simulink model "opti_debug"  (R2023a)
settings: Solver=FixedStepAuto  StartTime=0.0  StopTime=mdl.rt  RelTol=1e-3
values from neighbouring files (symbols this model uses):
  archived_Eul_XYZ = rst_Eul_XYZ.signals.values    [s4_run.m]    (also in step4_run_v1.m)
  archived_p_raw = rst_p_raw.signals.values    [s4_run.m]    (also in step4_run_v1.m)
  ctr = make_ext_tor_observer(rsim, mdl, ctr)    [s1_setup.m]    (also in setup_controller_with_functions.m = make_controller(); step1_setup.m; step1_setup_v1.m)
  ctr2 = ctr    [s1_setup.m]    (also in step1_setup.m; step1_setup_v1.m)
  lut = gen_lut    [s1_setup.m]    (also in thrust2voltage_lut_20230809.mat = ; thrust2voltage_lut_20230829.mat = )
  mdl = make_model(mdl,rsim)    [s1_setup.m]    (also in setup_controller_with_functions.m = make_model(flight_time); step1_setup.m; step1_setup_v1.m = make_model(flight_time,rsim))
  rbt = make_robot    [s1_setup.m]    (also in setup_controller_with_functions.m = make_robot(); step1_setup.m; step1_setup_v1.m)
  rbt2 = rbt    [s1_setup.m]    (also in step1_setup.m; step1_setup_v1.m)
  rsim = make_robot_simulation()    [setup_controller_with_functions.m]    (also in step1_setup_v1.m = make_simulation(rbt,mdl,rsim))
  sen = make_sensor(mdl,rsim)    [s1_setup.m]
  som = make_somersault(mdl, rsim)    [s1_setup.m]    (also in step1_setup.m)
  Time = logsout.LiveStreamSignals.getElement('voltage').Values.Time    [old_step3_run_controller_v3.m]    (also in post_identify_actuation_response.m = yout(:,1); post_thrust_torque_coefficients.m = yout(:,1))
  traj = make_trajectory(ctr, mdl, rsim)    [s1_setup.m]    (also in step1_setup.m)
undefined symbols (not defined in the file or in its folder): DiscIntNeverNeededParam, Discrete, Standard_Devices, UDP_Protocol
libraries: simulink x27, dspfdesign x12, robotcorelib x7, sldrtlib x7, slrealtimeloglib x1, shared6dof x1, dspsrcs4 x1, uavutilslib x1, ctrlSharedLib x1, dspmathops x1
(part 4 of 4)

== system opti_debug/Signal generater/signal generator1/signal generator 3/get max voltage/SIgnalForRamp_binary ==
  note: Should output 1 or -1,
      | so signal ramps UP to 1
      | or DOWN to 0.
  In1 : Inport
  Add : Sum  Inputs=+-
  Compare To Zero : simulink/Logic and Bit Operations/Compare To Zero  relop=>  OutDataTypeStr=uint8  ZeroCross=off
  Constant : Constant
  Data Type Conversion : DataTypeConversion  OutDataTypeStr=double  SaturateOnIntegerOverflow=off  RndMeth=Floor
  Gain : Gain  Gain=2
  Out1 : Outport
  wires:
  In1/1 -> Compare To Zero/1
  Compare To Zero/1 -> Data Type Conversion/1
  Gain/1 -> Add/1
  Constant/1 -> Add/2
  Add/1 -> Out1/1
  Data Type Conversion/1 -> Gain/1

== system opti_debug/Signal generater/signal generator1/signal generator 3/square root of sine wave/Subsystem1 ==
  cos wave : Inport
  new_amplitude : Inport  Port=2
  Delay : Delay  DelayLength=1  InitialCondition=0
  Delay1 : Delay  InitialCondition=[0,0]
  Delay2 : Delay  DelayLength=1  InitialCondition=0
  MATLAB Function : MATLAB Function  TreatAsAtomicUnit=on  SystemSampleTime=mdl.T_high
  output : Outport
  wires:
  cos wave/1 -> Delay1/1, Delay/1, MATLAB Function/1(u1)
  MATLAB Function/1(output) -> output/1, Delay2/1
  Delay/1 -> MATLAB Function/2(u2)
  Delay2/1 -> MATLAB Function/5(old_amplitude)
  Delay1/1 -> MATLAB Function/3(u3)
  new_amplitude/1 -> MATLAB Function/4(new_amplitude)

== system opti_debug/Signal generater/signal generator1/signal generator 4/get max voltage/SIgnalForRamp_binary ==
  note: Should output 1 or -1,
      | so signal ramps UP to 1
      | or DOWN to 0.
  In1 : Inport
  Add : Sum  Inputs=+-
  Compare To Zero : simulink/Logic and Bit Operations/Compare To Zero  relop=>  OutDataTypeStr=uint8  ZeroCross=off
  Constant : Constant
  Data Type Conversion : DataTypeConversion  OutDataTypeStr=double  SaturateOnIntegerOverflow=off  RndMeth=Floor
  Gain : Gain  Gain=2
  Out1 : Outport
  wires:
  In1/1 -> Compare To Zero/1
  Compare To Zero/1 -> Data Type Conversion/1
  Gain/1 -> Add/1
  Constant/1 -> Add/2
  Add/1 -> Out1/1
  Data Type Conversion/1 -> Gain/1

== system opti_debug/Signal generater/signal generator1/signal generator 4/square root of sine wave/Subsystem1 ==
  cos wave : Inport
  new_amplitude : Inport  Port=2
  Delay : Delay  DelayLength=1  InitialCondition=0
  Delay1 : Delay  InitialCondition=[0,0]
  Delay2 : Delay  DelayLength=1  InitialCondition=0
  MATLAB Function : MATLAB Function  TreatAsAtomicUnit=on  SystemSampleTime=mdl.T_high
  output : Outport
  wires:
  cos wave/1 -> Delay1/1, Delay/1, MATLAB Function/1(u1)
  MATLAB Function/1(output) -> output/1, Delay2/1
  Delay/1 -> MATLAB Function/2(u2)
  Delay2/1 -> MATLAB Function/5(old_amplitude)
  Delay1/1 -> MATLAB Function/3(u3)
  new_amplitude/1 -> MATLAB Function/4(new_amplitude)

== matlab function opti_debug/Motor thrust to voltage mapping/Subsystem/MATLAB Function ==
  data: t input; enable output; mdl parameter
function enable = fcn(t, mdl)

if t > mdl.i_delay && t < (mdl.i_delay + mdl.flight_time)
    enable = 1;
else
    enable = 0;
end

end

== matlab function opti_debug/Archived data for rerun/MATLAB Function1 ==
  data: t input; y output; archived_data_ready parameter
function y = fcn(t,archived_data_ready)

t = floor(t);
y = archived_data_ready(t,1);

end

== matlab function opti_debug/Archived data for rerun/MATLAB Function2 ==
  data: t input; y output; archived_p_raw parameter; archived_Eul_XYZ parameter
function y = fcn(t,archived_p_raw,archived_Eul_XYZ)

y = zeros(6,1);

t = floor(t);
y(1:3,1) = archived_p_raw(t,1:3)';
y(4:6,1) = archived_Eul_XYZ(t,1:3)';

end

== matlab function opti_debug/Control scheme/attitude and thrust controller/Subsystem/MATLAB Function ==
  data: time input; en_int output; ctr parameter; mdl parameter
function en_int = fcn(time, ctr, mdl)

    if ctr.takeoff.en
        wait_time = ctr.takeoff.time;
    else
        wait_time = 0;
    end
    
    if time > (mdl.i_delay + wait_time) && ctr.integral.en
        en_int = 1;
    else 
        en_int = 0;
    end

end

== matlab function opti_debug/Signal generater/signal generator1/signal generator 1/square root of sine wave/Subsystem1/MATLAB Function ==
  data: u1 input; output output; u2 input; u3 input; new_amplitude input; old_amplitude input
function output  = fcn(u1, u2, u3, new_amplitude, old_amplitude)

if u2 < u1 && u2 < u3
    output = new_amplitude;
else
    output = old_amplitude;
end

    
end

== matlab function opti_debug/Signal generater/signal generator1/signal generator 2/square root of sine wave/Subsystem1/MATLAB Function ==
  data: u1 input; output output; u2 input; u3 input; new_amplitude input; old_amplitude input
function output  = fcn(u1, u2, u3, new_amplitude, old_amplitude)

if u2 < u1 && u2 < u3
    output = new_amplitude;
else
    output = old_amplitude;
end

    
end

== matlab function opti_debug/Signal generater/signal generator1/signal generator 3/square root of sine wave/Subsystem1/MATLAB Function ==
  data: u1 input; output output; u2 input; u3 input; new_amplitude input; old_amplitude input
function output  = fcn(u1, u2, u3, new_amplitude, old_amplitude)

if u2 < u1 && u2 < u3
    output = new_amplitude;
else
    output = old_amplitude;
end

    
end

== matlab function opti_debug/Signal generater/signal generator1/signal generator 4/square root of sine wave/Subsystem1/MATLAB Function ==
  data: u1 input; output output; u2 input; u3 input; new_amplitude input; old_amplitude input
function output  = fcn(u1, u2, u3, new_amplitude, old_amplitude)

if u2 < u1 && u2 < u3
    output = new_amplitude;
else
    output = old_amplitude;
end

    
end

== matlab function opti_debug/State filters/IMU orientation/Subsystem2/Rotation Matrix ==
  data: euler_angles input; R output
function R = fcn(euler_angles)
%#codegen

eu_x = euler_angles(1);
eu_y = euler_angles(2);
eu_z = euler_angles(3);

R = [cos(eu_y)*cos(eu_z); -cos(eu_y)*sin(eu_z); sin(eu_y); ...
    cos(eu_x)*sin(eu_z)+sin(eu_x)*sin(eu_y)*cos(eu_z); cos(eu_x)*cos(eu_z)-sin(eu_x)*sin(eu_y)*sin(eu_z); -sin(eu_x)*cos(eu_y); ...
    sin(eu_x)*sin(eu_z)-cos(eu_x)*sin(eu_y)*cos(eu_z); sin(eu_x)*cos(eu_z)+cos(eu_x)*sin(eu_y)*sin(eu_z); cos(eu_x)*cos(eu_y)];


end

% R is 9x1

% Pakpong was using "XYZ" convention, which seems to be the same as Vicon

== matlab function opti_debug/State filters/range finder altitude estimator/motor thrust inverse mapping  ==
  data: sat_tor_thru input; total_thrust output; rbt parameter; mdl parameter
function total_thrust  = fcn(sat_tor_thru,rbt, mdl)

persistent time
if isempty(time); time = 0; end

thrust_in_N = sat_tor_thru(4);

if thrust_in_N > 0 && time > mdl.i_delay + 0.01
    total_thrust = thrust_in_N - mdl.g*rbt.m; 
else
    total_thrust = 0;
end

time = time + mdl.T;


end

== matlab function opti_debug/State filters/IMU orientation/Subsystem2/Rotation Matrix3 ==
  data: R input; Rdot input; w output
function w  = fcn(R,Rdot)
%#codegen
w = zeros(3,1);
w(1) = R(3)*Rdot(2) + R(6)*Rdot(5) + R(9)*Rdot(8);
w(2) = R(1)*Rdot(3) + R(4)*Rdot(6) + R(7)*Rdot(9);
w(3) = R(2)*Rdot(1) + R(5)*Rdot(4) + R(8)*Rdot(7);

% w = R^T * dot(R)

end

== matlab function opti_debug/State filters/IMU orientation/Subsystem2/MATLAB Function ==
  data: Eul_in input; R_dot output; mdl parameter
function R_dot  = fcn(Eul_in, mdl)

persistent  R_old R_dot_old dt

if isempty(dt); dt = 0; end
if isempty(R_old); R_old = zeros(9,1); end
if isempty(R_dot_old); R_dot_old = zeros(9,1); end

% Euler angle
eu_x = Eul_in(1);
eu_y = Eul_in(2);
eu_z = Eul_in(3);

% == WARNING == This is Pakpong's convention
R = [cos(eu_y)*cos(eu_z); -cos(eu_y)*sin(eu_z); sin(eu_y); ...
    cos(eu_x)*sin(eu_z)+sin(eu_x)*sin(eu_y)*cos(eu_z); cos(eu_x)*cos(eu_z)-sin(eu_x)*sin(eu_y)*sin(eu_z); -sin(eu_x)*cos(eu_y); ...
    sin(eu_x)*sin(eu_z)-cos(eu_x)*sin(eu_y)*cos(eu_z); sin(eu_x)*cos(eu_z)+cos(eu_x)*sin(eu_y)*sin(eu_z); cos(eu_x)*cos(eu_y)];


if R_old(3) == R(3) && R_old(6) == R(6)
    dt    = dt + mdl.T_high;
    R_dot = R_dot_old;
else
    dt    = dt + mdl.T_high;
    R_dot = (R - R_old)/dt;

    dt    = 0;
    R_old = R;
    R_dot_old = R_dot;
end

end

== matlab function opti_debug/State filters/optical flow position estimator/MATLAB Function ==
  data: R input; z input; distance output
function distance  = fcn(R,z)
z1=0;
R3 = R(:,3)/norm(R(:,3));
distance = (z+z1)/dot([0;0;1],R3);
end

== matlab function opti_debug/Motor thrust to voltage mapping/back mapping from sat volt to torque-thrust/power_distribution_1 ==
  data: motor_thrust input; torque_thrust output; rbt parameter
function torque_thrust  = fcn(motor_thrust, rbt)

% motor_thrust is in mgf
torque_x_mgfm = (- motor_thrust(1) + motor_thrust(2) ...
                 + motor_thrust(3) - motor_thrust(4)) * rbt.lt; % (mgf*m)
torque_y_mgfm = (- motor_thrust(1) - motor_thrust(2) ...
                 + motor_thrust(3) + motor_thrust(4)) * rbt.ld; % (mgf*m)
thrust_mgf    = (+ motor_thrust(1) + motor_thrust(2) ...
                 + motor_thrust(3) + motor_thrust(4)); % (mgf)        

% convert mgf to N (mgf*m & N*m)
torque = [torque_x_mgfm; torque_y_mgfm; 0] * 9.81e-6; %(N*m)
thrust = thrust_mgf * 9.81e-6; % (N)

torque_thrust = [torque; thrust];

% ==== original code ====
% r = torque(1) / roll_arm;
% p = torque(2) / pitch_arm; % (mgf) = (mgf*m) / (m)
% 
% att = [
%     - r - p;
%     + r - p;
%     + r + p;
%     - r + p]; % (mgf)
% 
% min_t = min(att);
% 
% if (thrust < - min_t)
%     thrust = - min_t; 
% end
%     
% m1 = thrust + att(1); % (mgf)
% m2 = thrust + att(2); % (mgf)
% m3 = thrust + att(3); % (mgf)
% m4 = thrust + att(4); % (mgf)
% 
% 
% motors_thrust = [m1; m2; m3; m4]; % (mgf)
% 
% return;
end

== matlab function opti_debug/State filters/optical flow position estimator/opt2vel ==
  data: opt input; opt_vx output; distance input; opt_vy output; sen parameter
function [opt_vx,opt_vy] = opt2vel(opt,distance, sen)

    opti_gain_x =  distance * sen.opt.k;
    opti_gain_y = -distance * sen.opt.k;
    opt_vx      =  opt(1) * opti_gain_x;
    opt_vy      =  opt(2) * opti_gain_y;

end

== matlab function opti_debug/State filters/optical flow position estimator/omegaCompensate ==
  data: opt_vx input; vx output; opt_vy input; omega input; distance input; vy output
function [vx,vy] = omegaCompensate(opt_vx,opt_vy,omega,distance)

    vx = opt_vx + distance*omega(2);
    vy = opt_vy - distance*omega(1);

end

== matlab function opti_debug/State filters/Safety check/MATLAB Function ==
  data: keep_flying input; en_in input; en_out output size=1; cum_in input; cum_out output size=1; ctr parameter; mdl parameter
function [en_out, cum_out] = fcn(keep_flying, en_in, cum_in, ctr, mdl)

if keep_flying == 0
    cum_out = cum_in + mdl.T;
else
    cum_out = 0;
end

if cum_out > ctr.safety.T || en_in == 0
    en_out = 0;
else 
    en_out = 1;
end

end

== matlab function opti_debug/State filters/Safety check/envelope check ==
  data: x input; en output; y input; z input; ctr parameter
function en  = fcn(x,y,z, ctr)

if abs(x)>ctr.safety.enableZone.xmax || abs(y)>ctr.safety.enableZone.ymax || abs(z)>ctr.safety.enableZone.zmax
    en = 0;
else
    en = 1;
end

end

== matlab function opti_debug/State filters/Safety check/voltage check ==
  data: voltage input; en output; ctr parameter
function en  = fcn(voltage, ctr)

    if sum(voltage > ctr.safety.volt) > 0
        en = 0;
    else
        en = 1;
    end

end

== matlab function opti_debug/State filters/range finder altitude estimator/MATLAB Function ==
  data: z input; z_compensated output; R input
function z_compensated  = fcn(z,R)

R3 = R(:,3)/norm(R(:,3));
z_compensated = z*dot([0;0;1],R3);
end

== matlab function opti_debug/State filters/range finder altitude estimator/MATLAB Function1 ==
  data: y input; u input; x_hat_new output; mdl parameter; rbt parameter
function x_hat_new = fcn(y, u, mdl, rbt)

    persistent time x_hat_old 
    if isempty(time); time = 0; end
    if isempty(x_hat_old); x_hat_old = [y; 0;]; end

    A = [0 1;
         0 0;];
    B = [0; 1/rbt.m];
    C = [1 0];

    L = [12; 20];

    x_hat_dot = A*x_hat_old + B*u + L*(y - C*x_hat_old);

    x_hat_new = x_hat_old + mdl.T_high * x_hat_dot;


    x_hat_old = x_hat_new;
    
    time = time + mdl.T_high;

end

== matlab function opti_debug/State filters/Safety check/MATLAB Function1 ==
  data: z input; y output; sen parameter
function y = fcn(z, sen)

    persistent z_zero_count
    
    if isempty(z_zero_count); z_zero_count = 0; end
    
    if z == 0
        z_zero_count = z_zero_count +1;
    end
    
    y = 1;
    
    if z_zero_count > sen.rgf.safety.count
        y = 0;
    end

end

== matlab function opti_debug/State filters/optical flow position estimator/condition optical flow ==
  data: u input; y output; sen parameter
function y = fcn(u, sen)

    if abs(u(1)) < sen.opt.threshold
        u(1) = 0;
    end
    if abs(u(2)) < sen.opt.threshold
        u(2) = 0;
    end
    y = u;

end

== matlab function opti_debug/State filters/optical flow position estimator/MATLAB Function1 ==
  data: vel_new input; ischange input; p_new output; mdl parameter
function p_new = fcn(vel_new,ischange, mdl)

    persistent time p_old vel_old time_old is_first
    if isempty(time); time = 0; end
    if isempty(time_old); time_old=0;end
    if isempty(p_old); p_old =[0;0]; end
    if isempty(vel_old); vel_old=[0;0]; end
    if isempty(is_first); is_first=1; end
    time = time + mdl.T_high;
    if abs(ischange)>eps
       if is_first==0
        p_new=p_old+(vel_new+vel_old)/2*(time-time_old);
        p_old=p_new;
       else
        is_first=0;
        p_new=p_old;
       end
        vel_old=vel_new;
        time_old=time;
    else
        p_new=p_old;
    end

end

== matlab function opti_debug/motor thrust mapping ==
  data: torque input; motors_thrust output; total_thrust input; rbt parameter
function motors_thrust = fcn(torque, total_thrust, rbt)

% torque in mgf*m
% total_thrust in mgf

% thrust of each unit
thrust = total_thrust/4;

% get force from body x/y axis torque  (consider moment arm)
r = torque(1) / rbt.lt / 4; % force on each unit (mgf)
p = torque(2) / rbt.ld / 4; % force on each unit (mgf)

% map force to each unit
att = [
    - r - p;
    + r - p;
    + r + p;
    - r + p];

% prioritize attitude over thrust
min_att  = min(att);
if (thrust < - min_att)
    thrust = - min_att; 
end

% map thrust and torque to each unit 
m1 = thrust + att(1);
m2 = thrust + att(2);
m3 = thrust + att(3);
m4 = thrust + att(4);

% create vector
motors_thrust = [m1; m2; m3; m4];

return;
end

== matlab function opti_debug/Control scheme/adaptive setpoint rd ==
  data: r input; rd output size=3; rd_d output size=3; rd_dd output size=3; rd_ddd output size=3; rd_dddd output size=3; init_r_out output size=3; time input; init_r_in input; id_in input; ctr2 parameter; mdl parameter; id_out output size=1; traj parameter
function [rd,rd_d,rd_dd,rd_ddd,rd_dddd,init_r_out, id_out] = fcn(r, time, init_r_in, id_in, ctr2, mdl, traj)

    % This function defines desired setpoint for the model-based controller

    persistent id init_r
    
    if isempty(id) 
        id = 1;
    else
        id = id +1;
    end

    if isempty(init_r) 
        init_r = zeros(3,1);
    end
    
    % Initialize output variables
    rd      = zeros(3,1); % postion
    rd_d    = zeros(3,1); % velocity
    rd_dd   = zeros(3,1); % acceleration
    rd_ddd  = zeros(3,1); % jerk
    rd_dddd = zeros(3,1); % snap

    % Get initial position of the robot
    if time < mdl.i_delay
        init_r_out = r(:);
        init_r = r(:);
    else
        init_r_out = init_r_in(:);
    end

    % Update id
    id_in   = floor(id_in);
    id_out  = id_in + 1;
    
    if ~traj.en
    
        % == No trajectory following (just takeoff and landing) ==
        rd = [init_r(1) + ctr2.setpoint.x;...
              init_r(2) + ctr2.setpoint.y;...
              init_r(3) + ctr2.setpoint.z];

        init_height    = init_r(3) + 0.003;
        init_height_to = init_r(3) + 0.004;
        
        % befor takeoff
        if time <= mdl.i_delay+0.03
            rd   = [init_r(1) + ctr2.setpoint.x;...
                    init_r(2) + ctr2.setpoint.y;...
                    init_height_to];
        end
        
        % takeoff
        if ctr2.takeoff.en
            if time > mdl.i_delay+0.03 && time < (mdl.i_delay+0.03+ctr2.takeoff.time)
                
                % rd_z (desired position)
                rd_z = init_height_to + (((init_r(3) + ctr2.setpoint.z-init_height_to)/ctr2.takeoff.time)*(time-mdl.i_delay-0.03));
                if rd_z > init_r(3) + ctr2.setpoint.z
                    rd_z = init_r(3) + ctr2.setpoint.z;
                end
                rd(3)  = rd_z;
                
                % rd_d_z (desired velocity)
                rd_d_z = ((init_r(3) + ctr2.setpoint.z-init_height_to)/ctr2.takeoff.time);
                rd_d   = [rd_d(1); rd_d(2); rd_d_z];
                
            end
        end
        
        % planned landing 
        if ctr2.landing.en
            if time > ((mdl.i_delay+mdl.flight_time)-ctr2.landing.time)
                
                % rd_z (desired position)
                rd_z = init_r(3) + ctr2.setpoint.z-(((init_r(3) + ctr2.setpoint.z-init_height)/ctr2.landing.time)*(time-(mdl.i_delay+mdl.flight_time)+ctr2.landing.time));
                if rd_z < init_height
                    rd_z = init_height;
                end
                rd(3)  =  rd_z;
                
                % rd_d_z (desired velocity)
                rd_d_z = (init_height-ctr2.setpoint.z-init_r(3))/ctr2.landing.time;
                rd_d   = [rd_d(1); rd_d(2); rd_d_z];
                
            end
        end

    else

        % == use pre-defined trajectory ==
       
        % use predefined trajectory
        if traj.en
            rd      = init_r + traj.rd(1:3,id);
            rd_d    = traj.rd_d(1:3,id);
            rd_dd   = traj.rd_dd(1:3,id);
            rd_ddd  = traj.rd_ddd(1:3,id);
            rd_dddd = traj.rd_dddd(1:3,id);
        end

    end



end

% somersault
% if som.en
%     if time > som.t_start + som.t_rise + som.t_acc + som.t_dcc + som.t_rec
%         % % afterwards 
%         %dt = som.t_start + som.t_rise + som.t_acc + som.t_dcc + som.t_rec - time;
%         %rd = rd + dt*(r-rd);
%     elseif time > som.t_start + som.t_rise + som.t_acc + som.t_dcc
%         % recovery
%         dt = som.t_start + som.t_rise + som.t_acc + som.t_dcc + som.t_rec - time;
%         rd = rd + (dt/som.t_rec)*(r-rd);
%         rd_d = rd_d + 0.5*(dt/som.t_rec)*(r_d-rd_d);
%         rd(1) = min(max(rd(1),-0.25),0.25); % 25 cm envelope
%         rd(2) = min(max(rd(2),-0.25),0.25); % 25 cm envelope
%         rd(3) = max(rd(3),0.02); % min altitude setpoint.
%     end
% end

== matlab function opti_debug/Control scheme/attitude and thrust controller/Controller ==
  data: r input; torque_x output size=1; r_dot input; r_dotdot input; R input; Omega input; rd input; rd_d input; rd_dd input; rd_ddd input; rd_dddd input; ext_torq input; int_tf input; time input; ctr parameter; rbt parameter; torque_y output size=1; torque_z output size=1; F output; torque_gyro_x output; torque_gyro_y output; mdl parameter; att_e output; alt_e output; traj parameter; som parameter; state output; R33 output; eulx output; eulZYX output
function [torque_x, torque_y, torque_z, F, torque_gyro_x, torque_gyro_y, att_e, alt_e, state, R33 ,eulx, eulZYX] = fcn(r, r_dot, r_dotdot, R, Omega, rd,rd_d,rd_dd,rd_ddd,rd_dddd, ext_torq, int_tf, time, ctr, rbt, mdl, traj, som)
    
% ==================================
% ==== preliminary =================
% ==================================
    
    % persistent variables
    persistent id som_state t_fall t_dec z_setpoint t_hover t_rot_acc t_safe
    if isempty(id); id = 1; else; id = id +1; end
    if isempty(som_state); som_state = 0; end
    if isempty(t_fall); t_fall = 0; end
    if isempty(t_dec); t_dec = 0; end
    if isempty(z_setpoint); z_setpoint = rd(3); end
    if isempty(t_hover); t_hover = 0; end
    if isempty(t_rot_acc); t_rot_acc = 0; end
    if isempty(t_safe); t_safe = 0; end

    % get compact notation
    R1     = R(:,1);
    R2     = R(:,2);
    R3     = R(:,3);
    wx     = Omega(1);
    wy     = Omega(2);
    wz     = Omega(3);
    w      = Omega(:);
    Dr     = r-rd;
    Dr_dot = r_dot-rd_d;
    J      = diag([rbt.ixx, rbt.iyy, rbt.izz]);
    eulZYX = rotm2eul(R,'ZYX');
    eulZXY = rotm2eul(R,'ZXY');
    eulx   = eulZYX(3);
    euly   = eulZXY(3);

    if euly > 2
        euly = euly - (2*pi);
    end

    if eulx > 2
        eulx = eulx - (2*pi);
    end

% ==================================
% ==== somersault state ============
% ==================================
    if som.en

        % som_state == 0 is nominal hovering controller

        if som.testing.en
            
            % get into no thrust state
            if som_state == 1 && r_dot(3) >= som.threshold.z_dot.acc
                som_state = 7;

            elseif som_state == 1 && r(3) >= som.testing.z
                som_state = 5;

            % get into translational deceleration
            elseif som_state == 7 && t_fall >= som.testing.drop_time
                som_state = 4;
            end

        end
        
        % get into translational acceleration
        if som_state == 0 && time >= som.t.acc % && r_dot(3) < som.threshold.z_dot.acc
            som_state = 1;
        
        % get into norminal controller if it goes too high
        elseif som_state == 1 && r(3) >= 0.30
            som_state = 5;

        % get into flip acceleration
        elseif som_state == 1 && r_dot(3) >= som.threshold.z_dot.acc
            som_state = 2;

        % get into flip deceleration
        % elseif som_state == 2 && eulx < 0 && eulx >= som.threshold.down.eulx && R(3,3) <= som.threshold.down.R33
        elseif som_state == 2 && eulx >= som.threshold.down.euly && R(3,3) <= som.threshold.down.R33 && t_rot_acc > som.threshold.t_rot_acc
            som_state = 3;

        % get into translational deceleration
        elseif som_state == 3 && wx < som.threshold.wy
            som_state = 3.5;

        % get into translational deceleration
        elseif som_state == 3.5 && R(3,3) >= som.threshold.up.R33 && wx < som.threshold.up.wy
            som_state = 4;

        % get low-gain hovering controller
        elseif som_state == 4 && r_dot(3) > som.threshold.z_dot.dec && t_dec > 0.2
            som_state = 4.5;

        % get into nominal hovering controller
        elseif som_state == 4.5 && t_dec > 0.5
            som_state = 5;
            if r(3) > rd(3)
                z_setpoint = r(3);
            else
                z_setpoint = rd(3);
            end

        % get into safety mode
        elseif som_state == 1 && (r(3) >= 0.30 || r(3) < 0.02) 
            som_state = 5;

        end
    end


% ==================================
% ==== altitude controller =========
% ==================================
    if som.en
        if som_state == 5
            t_hover = t_hover + mdl.T;
            if t_hover > som.t_hover
                
            else
                rd(3) = z_setpoint;
            end
        end
    end
    
    % linear feedforward (for the tether weight)
    ffwd = mdl.g * max(0,rd(3)*ctr.gain.alfd);
    
    % desired net acceleration for the 2nd-order system (not taking r_dotdot)
    a_net = rd_dd(3) - ctr.gain.al1*( r_dot(3)-rd_d(3) ) - ctr.gain.al0*( r(3)-rd(3) );
    
    % gravity + net acceleration + integral term + feedforward
    a_w = mdl.g + a_net + int_tf(4) + ffwd + ctr.thrust_offset; % world frame

    % world to body frame
    a_b = a_w/R(3,3);

    % saturation
    a = max(min(a_b, mdl.g + 5), mdl.g - 3.0); % during hovering.

    % convert accelearation to Newton
    F = a*rbt.m;


% ==================================
% ==== lateral controller ==========
% ==================================

    % get thrust correction  
    acc_net_b     = 0;
    acc_net_dot_b = 0;

    if ctr.atmg.en
        acc_net_b     = traj.thrust_b(id); % thrust for aggresive traj
        acc_net_dot_b = traj.thrust_b_dot;
    end

    if som.en
        if som_state == 1 
            acc_net_b = (som.thrust.acc - mdl.g) * rbt.m; % accelerate at the predetermined value
        elseif som_state == 4 
            acc_net_b = (som.thrust.dec - mdl.g) * rbt.m; % decelerate at the predetermined value
        % elseif som_state == 5
        %     acc_net_b = (a-mdl.g) * rbt.m; 
        end
    end

    % set gain
    if som.en
        if som_state == 3
            ctr.gain.at3 = ctr.gain.at3 * som.gain.fact.st3.at3;
            ctr.gain.at2 = ctr.gain.at2 * som.gain.fact.st3.at2;
            ctr.gain.at1 = ctr.gain.at1 * som.gain.fact.st3.at1;
            ctr.gain.at0 = ctr.gain.at0 * som.gain.fact.st3.at0;
            ctr.torque_obs.factor.x = 0;
            ctr.torque_obs.factor.y = 0;
        elseif som_state == 4
            ctr.gain.at3 = ctr.gain.at3 * som.gain.fact.st4.at3;
            ctr.gain.at2 = ctr.gain.at2 * som.gain.fact.st4.at2;
            ctr.gain.at1 = ctr.gain.at1 * som.gain.fact.st4.at1;
            ctr.gain.at0 = ctr.gain.at0 * som.gain.fact.st4.at0;
            ctr.torque_obs.factor.x = 0;
            ctr.torque_obs.factor.y = 0;

        elseif som_state == 4.5
            ctr.gain.at3 = ctr.gain.at3 * som.gain.fact.st45.at3;
            ctr.gain.at2 = ctr.gain.at2 * som.gain.fact.st45.at2;
            ctr.gain.at1 = ctr.gain.at1 * som.gain.fact.st45.at1;
            ctr.gain.at0 = ctr.gain.at0 * som.gain.fact.st45.at0;
            ctr.torque_obs.factor.x = 0;
            ctr.torque_obs.factor.y = 0;
        end
    end

   
    % % get desired angular accelaration
    des_wx_dot = (- dot(R2,rd_dddd)  ...
                  - ctr.gain.at3*( (mdl.g+max(-0.1,acc_net_b))*wx+dot(R2,rd_ddd) )  ...
                  - ctr.gain.at2*( dot(R2,mdl.g*[0;0;1]+rd_dd) )  ...
                  + ctr.gain.at1*( dot(R2,Dr_dot) )  ...
                  + ctr.gain.at0*( dot(R2,Dr) ) ) ...
                  /((mdl.g+max(-0.5,acc_net_b*ctr.gain.atmg.factor.x))); % 

    des_wy_dot = (+ dot(R1,rd_dddd)  ...
                  - ctr.gain.at3*( (mdl.g+max(-0.1,acc_net_b))*wy-dot(R1,rd_ddd) )  ...
                  - ctr.gain.at2*( dot(R1,-mdl.g*[0;0;1]-rd_dd) )  ...
                  - ctr.gain.at1*( dot(R1,Dr_dot) )  ...
                  - ctr.gain.at0*( dot(R1,Dr) )) ...
                  / ((mdl.g+max(-0.5,acc_net_b*ctr.gain.atmg.factor.x))); % + ...

    % gyropscopic effect (might be noisy)
    torque_gyro = J*[des_wx_dot; des_wy_dot; 0] + cross(w,J*w);

    % just moment of inertia
    torque = J*[des_wx_dot; des_wy_dot; 0];

    % get torque
    torque_x = torque(1) - ext_torq(1)*ctr.torque_obs.factor.x + int_tf(1) + ctr.torque_offset.x;
    torque_y = torque(2) - ext_torq(2)*ctr.torque_obs.factor.y + int_tf(2) + ctr.torque_offset.y;
    torque_z = 0; % no yaw control

    torque_gyro_x = torque_gyro(1) - ext_torq(1)*ctr.torque_obs.factor.x + int_tf(1) + ctr.torque_offset.x;
    torque_gyro_y = torque_gyro(2) - ext_torq(2)*ctr.torque_obs.factor.y + int_tf(2) + ctr.torque_offset.y;


% ==================================
% ==== intergral error =============
% ==================================

    % attitude error
    att_e = [dot(R2,Dr);-dot(R1,Dr);0];

    % altitude error
    alt_e = -( r(3)-rd(3) )/R(3,3);


% ==================================
% ==== somersault torque/thrsut ====
% ==================================

    if som.en
        
        % translational acceleration
        if som_state == 1
            F = som.thrust.acc * rbt.m;
            alt_e = 0;

        % flip acceleration
        elseif som_state == 2

            % cumulate time
            t_rot_acc = t_rot_acc + mdl.T;

            % rotate in x-axis
            torque_x = som.tor_y.acc + int_tf(1) + ctr.torque_offset.x;
            torque_y = 0;

            % % rotate in y-axis
            % torque_x = 0;
            % torque_y = som.tor_y.acc + int_tf(2) + ctr.torque_offset.y;

            F = 0;
            alt_e = 0;
            att_e = zeros(3,1);

        % flip deceleration
        elseif som_state == 3

            % == Rotate in x-axis ==
            torque_x = som.tor_y.dec;


            % % == Rotate in y-axis ==
            
            % if wy > som.threshold.wy
            %     torque_y = som.tor_y.dec;
            % else
            %     torque_y = + (0-euly) * som.tor_y.gain.dec.p ...
            %                + (0-wy) * som.tor_y.gain.dec.d;
            % end

            F = 0;
            alt_e = 0;
            att_e = zeros(3,1);

            t_safe = t_safe + mdl.T;

            if t_safe > 0.3
                F = 0;
                torque_x = 0;
                torque_y = 0;
            end

        % flip deceleration
        elseif som_state == 3.5

            % == Rotate in x-axis ==
            torque_x = + (0-eulx) * som.tor_y.gain.dec.p ...
                       + (0-wx) * som.tor_y.gain.dec.d;

            % % == Rotate in y-axis ==
            
            % if wy > som.threshold.wy
            %     torque_y = som.tor_y.dec;
            % else
            %     torque_y = + (0-euly) * som.tor_y.gain.dec.p ...
            %                + (0-wy) * som.tor_y.gain.dec.d;
            % end

            F = 0;
            alt_e = 0;
            att_e = zeros(3,1);

            t_safe = t_safe + mdl.T;

            if t_safe > 0.3
                F = 0;
                torque_x = 0;
                torque_y = 0;
            end


        % translational deceleration
        elseif som_state == 4
            F = som.thrust.dec * rbt.m;
            t_dec = t_dec + mdl.T;
            alt_e = 0;

        % low gain hovering
        elseif som_state == 4.5
            F = mdl.g * rbt.m;
            t_dec = t_dec + mdl.T;
            alt_e = 0;

        % safety feature
        elseif som_state == 5 && R(3,3) < -0.2
            F = 0;
            torque_x = 0;
            torque_y = 0;

        elseif som_state == 7
            F = 0;
            t_fall = t_fall + mdl.T;

        end

    end
    
% torque_gyro = ones(3,1);
state = som_state;
R33 = R(3,3);

 end

== matlab function opti_debug/State filters/Vicon orientation/Subsystem5/Rotation Matrix ==
  data: euler_angles input; R output
function R = fcn(euler_angles)
%#codegen

eu_x = euler_angles(1);
eu_y = euler_angles(2);
eu_z = euler_angles(3);

R = [cos(eu_y)*cos(eu_z); -cos(eu_y)*sin(eu_z); sin(eu_y); ...
    cos(eu_x)*sin(eu_z)+sin(eu_x)*sin(eu_y)*cos(eu_z); cos(eu_x)*cos(eu_z)-sin(eu_x)*sin(eu_y)*sin(eu_z); -sin(eu_x)*cos(eu_y); ...
    sin(eu_x)*sin(eu_z)-cos(eu_x)*sin(eu_y)*cos(eu_z); sin(eu_x)*cos(eu_z)+cos(eu_x)*sin(eu_y)*sin(eu_z); cos(eu_x)*cos(eu_y)];


end

% R is 9x1

% Pakpong was using "XYZ" convention, which seems to be the same as Vicon

== matlab function opti_debug/Control scheme/attitude and thrust controller/External Torque Observer ==
  data: ext_torque_hat output; omega input; omega_hat output; torque_x input; torque_y input; ext_torque_hat input; omega_hat input; time input; ctr2 parameter; rbt2 parameter; mdl parameter
function [ext_torque_hat, omega_hat] = fcn(omega, torque_x, torque_y, ext_torque_hat, omega_hat, time, ctr2, rbt2, mdl)
    
omega_hat           = omega_hat(:);
ext_torque_hat      = ext_torque_hat(:);
J                   = diag([rbt2.ixx, rbt2.iyy, rbt2.izz]);
omega_cross_J_omega = cross(omega, J*omega);
x_hat_curr          = diag(ctr2.torque_obs.state_scaling)*[omega_hat(:); ext_torque_hat(:)];

% til = 20;

% if rbt2.til == 0
u              = diag(ctr2.torque_obs.input_scaling)*[torque_x - omega_cross_J_omega(1); torque_y - omega_cross_J_omega(2)];
y              = diag(ctr2.torque_obs.meas_scaling)*omega(1:2); 
x_hat_pred     = ctr2.torque_obs.A*x_hat_curr + ctr2.torque_obs.B(:, 1:2)*u; 
x_hat_next     = diag(ctr2.torque_obs.out_scaling)*(x_hat_pred + ctr2.torque_obs.L*(y - ctr2.torque_obs.C*x_hat_pred));
omega_hat      = x_hat_next(1:2,1);
ext_torque_hat = x_hat_next(3:4,1);
if time < mdl.i_delay
    omega_hat      = zeros(2,1);
    ext_torque_hat = zeros(2,1);
end
% else
%     u              = diag(ctr2.torque_obs.input_scaling)*[torque_x - omega_cross_J_omega(1); torque_y - omega_cross_J_omega(2); torque_z - omega_cross_J_omega(3)];
%     y              = diag(ctr2.torque_obs.meas_scaling)*omega(1:3); 
%     x_hat_pred     = ctr2.torque_obs.A*x_hat_curr + ctr2.torque_obs.B(:, 1:3)*u; 
%     x_hat_next     = diag(ctr2.torque_obs.out_scaling)*(x_hat_pred + ctr2.torque_obs.L*(y - ctr2.torque_obs.C*x_hat_pred));
%     omega_hat      = x_hat_next(1:3,1);
%     ext_torque_hat = x_hat_next(4:6,1);
%     if time < mdl.i_delay
%         omega_hat      = zeros(3,1);
%         ext_torque_hat = zeros(3,1);
%     end
% end



end

== matlab function opti_debug/Control scheme/attitude and thrust controller/Thrust Controller ==
  data: r input; F output size=1; r_dot input; r_dotdot input; R input; Omega input; rd input; rd_d input; rd_dd input; rd_ddd input; rd_dddd input; int_tf input; mdl parameter; ctr parameter; alt_e output size=1; rbt parameter
function [F, alt_e]  = fcn(r, r_dot, r_dotdot, R, Omega, rd,rd_d,rd_dd,rd_ddd,rd_dddd, int_tf, mdl, ctr, rbt)

    % initialize
    R33 = R(9); % body to world
    
    % linear feedforward (for the tether weight)
    ffwd = mdl.g * max(0,rd(3)*ctr.gain.alfd);
    
    % desired net acceleration for the 2nd-order system (not taking r_dotdot)
    a_net = rd_dd(3) - ctr.gain.al1*( r_dot(3)-rd_d(3) ) - ctr.gain.al0*( r(3)-rd(3) );
    
    % gravity + net acceleration + integral term + feedforward
    a_w = mdl.g + a_net + int_tf(4) + ffwd + ctr.thrust_offset;

    % world to body frame
    a_b = a_w/R33;

    % saturation
    a = max(min(a_b, mdl.g+4), mdl.g-4.0); % during hovering.

    % convert accelearation to Newton
    F = a*rbt.m;
    
    % get intergral error
    alt_e = -( r(3)-rd(3) )/R33;

    % somersault
    if som.en
        
        % accelerate at the predetermined value
        if time > som.t1 && <= som.t2
            F = som.acc * rbt.m; 

        % no thrust during flipping
        elseif time > som.t2 && time <= som.t3
            F = 0;
            

        end

        

    end

end

== matlab function opti_debug/Control scheme/attitude and thrust controller/Yaw Controller/MATLAB Function ==
  data: torq_ext input; torq_z input; torq_z output; ctr2 parameter; rbt2 parameter
function torq_z = fcn(torq_ext,torq_z,ctr2, rbt2)

if rbt2.til > 0
    if ctr2.yaw.dy.en == 0
%         torq_z = torq_z - torq_ext(3) * ctr2.torque_obs.factor.z;
    end
else
    torq_z = torq_z;
end

end

== matlab function opti_debug/Control scheme/attitude and thrust controller/Yaw Controller/desired yaw ==
  data: t input; id input; rd_yaw output; ctr2 parameter; index output; mdl parameter
function [rd_yaw, index] = fcn(t,id,ctr2,mdl)

if ctr2.yaw.dy.en
    
    if id > 1
        t_cum = sum(ctr2.yaw.dy.duration(1:id-1))+sum(ctr2.yaw.dy.trans(1:id-1));
    else
        t_cum = 0;
    end

    if t > mdl.i_delay + t_cum && t <= mdl.i_delay + t_cum + ctr2.yaw.dy.duration(id)
        rd_yaw = ctr2.yaw.dy.angle(id);
    elseif t > mdl.i_delay + t_cum + ctr2.yaw.dy.duration(id) && t < mdl.i_delay + t_cum + ctr2.yaw.dy.duration(id) + ctr2.yaw.dy.trans(id)
        rd_yaw = ctr2.yaw.dy.angle(id) + (ctr2.yaw.dy.angle(id+1)-ctr2.yaw.dy.angle(id))/ctr2.yaw.dy.trans(id)*(t-mdl.i_delay-t_cum-ctr2.yaw.dy.duration(id));
    elseif t >= mdl.i_delay + t_cum + ctr2.yaw.dy.duration(id) + ctr2.yaw.dy.trans(id)
        rd_yaw = ctr2.yaw.dy.angle(id+1);
        id = id + 1;
    else
        rd_yaw = 0;
    end

else
    
    rd_yaw = ctr2.setpoint.yaw;
    
end

index = id;
    
end

== matlab function opti_debug/Control scheme/observer/Rotaion/Rotation Matrix ==
  data: euler_angles input; R output
function R = fcn(euler_angles)
%#codegen

eu_x = euler_angles(1);
eu_y = euler_angles(2);
eu_z = euler_angles(3);

R = [cos(eu_y)*cos(eu_z); -cos(eu_y)*sin(eu_z); sin(eu_y); ...
    cos(eu_x)*sin(eu_z)+sin(eu_x)*sin(eu_y)*cos(eu_z); cos(eu_x)*cos(eu_z)-sin(eu_x)*sin(eu_y)*sin(eu_z); -sin(eu_x)*cos(eu_y); ...
    sin(eu_x)*sin(eu_z)-cos(eu_x)*sin(eu_y)*cos(eu_z); sin(eu_x)*cos(eu_z)+cos(eu_x)*sin(eu_y)*sin(eu_z); cos(eu_x)*cos(eu_y)];
% R is 1x9

== matlab function opti_debug/Control scheme/observer/Rotaion/Rotation Matrix1 ==
  data: R input; Rdot input; w output
function w  = fcn(R,Rdot)
%#codegen
w = zeros(3,1);
w(1) = R(3)*Rdot(2) + R(6)*Rdot(5) + R(9)*Rdot(8);
w(2) = R(1)*Rdot(3) + R(4)*Rdot(6) + R(7)*Rdot(9);
w(3) = R(2)*Rdot(1) + R(5)*Rdot(4) + R(8)*Rdot(7);

== matlab function opti_debug/Control scheme/saturation ==
  data: x_roll input; X_roll output size=1; y_pitch input; z_yaw input; Y_pitch output size=1; Z_yaw output size=1; F input; Force output size=1; ctr2 parameter
function [X_roll, Y_pitch, Z_yaw, Force] = fcn(x_roll, y_pitch, z_yaw, F, ctr2)


    X_roll = max(min(x_roll, ctr2.lim.taux), -ctr2.lim.taux);
    
    Y_pitch = max(min(y_pitch, ctr2.lim.tauy), -ctr2.lim.tauy);
    
    Z_yaw = max(min(z_yaw, ctr2.lim.tauz), -ctr2.lim.tauz);
    
    Force = F;

end

% F is already checked for saturation

  
% Thrust management
% thrust is not controlled during the flipping maneuver (the output here will be overridden in the mapping).

== matlab function opti_debug/State filters/Vicon orientation/Subsystem5/Rotation Matrix2 ==
  data: R input; Rdot input; w output
function w  = fcn(R,Rdot)
%#codegen
w = zeros(3,1);
w(1) = R(3)*Rdot(2) + R(6)*Rdot(5) + R(9)*Rdot(8);
w(2) = R(1)*Rdot(3) + R(4)*Rdot(6) + R(7)*Rdot(9);
w(3) = R(2)*Rdot(1) + R(5)*Rdot(4) + R(8)*Rdot(7);

% w = R^T * dot(R)

end

== matlab function opti_debug/State filters/Vicon orientation/Subsystem5/Rotation Matrix3 ==
  data: R input; Rdot input; w output
function w  = fcn(R,Rdot)
%#codegen
w = zeros(3,1);
w(1) = R(3)*Rdot(2) + R(6)*Rdot(5) + R(9)*Rdot(8);
w(2) = R(1)*Rdot(3) + R(4)*Rdot(6) + R(7)*Rdot(9);
w(3) = R(2)*Rdot(1) + R(5)*Rdot(4) + R(8)*Rdot(7);

% w = R^T * dot(R)

end

== matlab function opti_debug/Signal generater/signal generator1/signal generator 4/Subsystem/MATLAB Function ==
  data: u1 input; output output; u2 input; u3 input; new_amplitude input; old_amplitude input
function output  = fcn(u1, u2, u3, new_amplitude, old_amplitude)

if u2 < u1 && u2 < u3
    output = new_amplitude;
else
    output = old_amplitude;
end

    
end

== matlab function opti_debug/Signal generater/signal generator1/signal generator 3/Subsystem/MATLAB Function ==
  data: u1 input; output output; u2 input; u3 input; new_amplitude input; old_amplitude input
function output  = fcn(u1, u2, u3, new_amplitude, old_amplitude)

if u2 < u1 && u2 < u3
    output = new_amplitude;
else
    output = old_amplitude;
end

    
end

== matlab function opti_debug/Signal generater/signal generator1/signal generator 2/Subsystem/MATLAB Function ==
  data: u1 input; output output; u2 input; u3 input; new_amplitude input; old_amplitude input
function output  = fcn(u1, u2, u3, new_amplitude, old_amplitude)

if u2 < u1 && u2 < u3
    output = new_amplitude;
else
    output = old_amplitude;
end

    
end

== matlab function opti_debug/Signal generater/signal generator1/signal generator 1/original sine wave/Subsystem/MATLAB Function ==
  data: u1 input; output output; u2 input; u3 input; new_amplitude input; old_amplitude input
function output  = fcn(u1, u2, u3, new_amplitude, old_amplitude)

if u2 < u1 && u2 < u3
    output = new_amplitude;
else
    output = old_amplitude;
end

    
end
